simulink model "Encoder_Zynq_V25"  (R2021a)
settings: Solver=FixedStepDiscrete  StartTime=0.0  StopTime=SimulationsDauer  RelTol=1e-3
values from neighbouring files (symbols this model uses):
  f_ISR = 40e3    (= 40000)    [Script_Encoder_Zynq.m]
  IncPerTurn = 1024    [Script_Encoder_Zynq.m]
  inital_zero_speed_timeout = speed_timeout_in_s*f_fpga    (= 10000)    [Script_Encoder_Zynq.m]
  n_max = 6000    [Script_Encoder_Zynq.m]
  OmegaPerOverSampl = 500*((2*pi)/60)    (= 52.3598775598)    [Script_Encoder_Zynq.m]
  Periode = abs(1/Striche_pro_Sekunde)    [Script_Encoder_Zynq.m]
  Phase_Delay_A = Periode/8    [Script_Encoder_Zynq.m]
  Phase_Delay_B = -Periode/8    [Script_Encoder_Zynq.m]
  PolePair = 1    [Script_Encoder_Zynq.m]
  QuadratureFactor = 4    [Script_Encoder_Zynq.m]
  reciprocal_iterations = 3    [Script_Encoder_Zynq.m]
  T_50MHz = 1/f_50MHz    (= 1e-08)    [Script_Encoder_Zynq.m]
  T_mech = 1e-08    [Script_Encoder_Zynq.m]
undefined symbols (not defined in the file or in its folder): DiscIntNeverNeededParam, Newton, Raphson
libraries: hdlsllib x17, dspsrcs4 x3, simulink x2, dspswit3 x2, spsEdgeDetectorLib x2, simulink_extras x1, spspowerguiLib x1
(part 1 of 3)
settings Model: DataTypeOverride=Off  Creator=Wendel_ELSYS  LastModifiedBy=ga92wum
settings SolverCC: ConcurrentTasks=on  AlgebraicLoopSolver=TrustRegion  MinimalZcImpactIntegration=on
settings DataIOCC: LimitDataPoints=on  SaveFormat=Array
settings OptimizationCC: BlockReduction=off  ConditionallyExecuteInputs=off  DefaultParameterBehavior=Inlined  LifeSpan=inf
settings DebuggingCC: ReadBeforeWriteMsg=DisableAll  WriteAfterWriteMsg=DisableAll  WriteAfterReadMsg=DisableAll  AlgebraicLoopMsg=error  SingleTaskRateTransMsg=error  ParameterOverflowMsg=none  SFUnexpectedBacktrackingDiag=warning  SFNoUnconditionalDefaultTransitionDiag=warning  SFExecutionAtInitializationDiag=none  SFMachineParentedDataDiag=warning  ArithmeticOperatorsInVariantConditions=warning
settings HardwareCC: ProdBitPerPointer=32  ProdBitPerSizeT=32  ProdBitPerPtrDiffT=32  ProdLargestAtomicFloat=None  ProdIntDivRoundTo=Undefined  ProdEndianess=Unspecified  ProdWordSize=32  ProdHWDeviceType=ASIC/FPGA->ASIC/FPGA  ProdEqTarget=off
settings ModelReferenceCC: UpdateModelReferenceTargets=IfOutOfDate  PropagateSignalLabelsOutOfModel=off
settings SFSimCC: SFSimEcho=off  SimUseLocalCustomCode=off  CustomCodeUndefinedFunction=UseInterfaceOnly
settings RTWCC: RTWUseLocalCustomCode=off
settings CodeAppCC: StateflowObjectComments=on
settings GRTTargetCC: TargetLangStandard=C89/C90 (ANSI)
settings ConfigComp: CovMetricSettings=dw  CovSaveCumulativeToWorkspaceVar=on  CovSaveSingleToWorkspaceVar=on  CovExternalEMLEnable=off
settings SimscapeCC: SimscapeNormalizeSystem=off

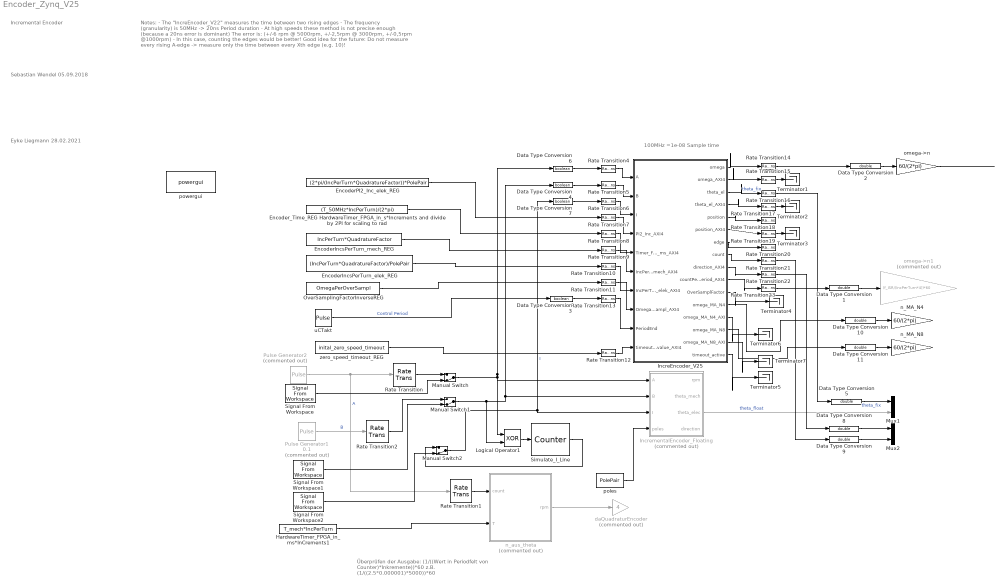
== system Encoder_Zynq_V25 ==
  note: 100MHz =1e-08 Sample time
  note: Überprüfen der Ausgabe:
      | (1/((Wert in Periodfelt von Counter)*Inkremente))*60
      | z.B. (1/((2.5*0.000001)*5000))*60
  note: Sebastian Wendel
      | 05.09.2018
  note: Notes:
      | - The "IncreEncoder_V22" measures the time between two rising edges
      | - The frequency (granularity) is 50MHz -> 20ns Period duration
      | - At high speeds these method is not precise enough (because a 20ns error is dominant)
      | The error is: (+/-6 rpm @ 5000rpm, +/-2,5rpm @ 3000rpm, +/-0,5rpm @1000rpm)
      | - In this case, counting the edges would be better!
      |
      | Good idea for the future: Do not measure every rising A-edge
      | -> measure only the time between every Xth edge (e.g. 10)!
  note: Incremental Encoder
  note: Eyke Liegmann
      | 28.02.2021
  Data Type Conversion{1..2,5,8..11} (7 alike) : DataTypeConversion  OutDataTypeStr=double
  Data Type Conversion{3..4,6..7} (4 alike) : DataTypeConversion  OutDataTypeStr=boolean
  "EncoderIncsPerTurn_elek_REG " : Constant  Value=(IncPerTurn*QuadratureFactor)/PolePair  OutDataTypeStr=fixdt(0,16,0)  SampleTime=T_mech
  EncoderIncsPerTurn_mech_REG : Constant  Value=IncPerTurn*QuadratureFactor  OutDataTypeStr=fixdt(0,16,0)  SampleTime=T_mech
  EncoderPI2_Inc_elek_REG : Constant  Value=(2*pi/(IncPerTurn*QuadratureFactor))*PolePair  OutDataTypeStr=fixdt(0,24,24)  SampleTime=T_mech
  Encoder_Time_REG HardwareTimer_FPGA_in_s*Increments and divide by 2PI for scaling to rad : Constant  Value=(T_50MHz*IncPerTurn)/(2*pi)  OutDataTypeStr=fixdt(0,32,32)  SampleTime=T_mech
  HardwareTimer_FPGA_in_ms*InCrements1 : Constant  Value=T_mech*IncPerTurn  OutDataTypeStr=double  SampleTime=T_mech
  IncreEncoder_V25 : Subsystem  TreatAsAtomicUnit=on
  IncrementalEncoder_Floating : Subsystem  Commented=on
  Logical Operator1 : Logic  Operator=XOR  AllPortsSameDT=off  OutDataTypeStr=boolean
  Manual Switch : ManualSwitch  CurrentSetting=0
  Manual Switch1 : ManualSwitch  CurrentSetting=0
  Manual Switch2 : ManualSwitch  CurrentSetting=0
  Mux1 : Mux  Inputs=2
  Mux2 : Mux  Inputs=2
  OverSamplingFactorInverseREG : Constant  Value=OmegaPerOverSampl  OutDataTypeStr=fixdt(1,24,11)  SampleTime=T_mech
  Pulse Generator1 0.1 : DiscretePulseGenerator  Commented=on  PulseType=Time based  Period=Periode  PulseWidth=50  PhaseDelay=Phase_Delay_B  SampleTime=T_mech  VectorParams1D=off
  Pulse Generator2 : DiscretePulseGenerator  Commented=on  PulseType=Time based  Period=Periode  PulseWidth=50  PhaseDelay=Phase_Delay_A  SampleTime=T_mech  VectorParams1D=off
  Rate Transition{,1..2,14..23} (13 alike) : RateTransition  Deterministic=off  OutPortSampleTime=T_mech
  Rate Transition{4..13} (10 alike) : RateTransition  Deterministic=off  OutPortSampleTime=T_50MHz
  Signal From Workspace : dspsrcs4/Signal From Workspace  X=A_ila  Ts=T_mech  nsamps=1  OutputAfterFinalValue=Setting to zero  ignoreOrWarnInputAndFrameLengths=off  OutputFrames=off
  Signal From Workspace1 : dspsrcs4/Signal From Workspace  X=B_ila  Ts=T_mech  nsamps=1  OutputAfterFinalValue=Setting to zero  ignoreOrWarnInputAndFrameLengths=off  OutputFrames=off
  Signal From Workspace2 : dspsrcs4/Signal From Workspace  X=I_ila  Ts=T_mech  nsamps=1  OutputAfterFinalValue=Setting to zero  ignoreOrWarnInputAndFrameLengths=off  OutputFrames=off
  Simulate_I_Line : dspswit3/Counter  Direction=Up  CountEvent=Either edge  CounterSize=User defined  MaxCount=IncPerTurn*4  InitialCount=0  Output=Hit  HitValue=IncPerTurn*4  ResetInput=off  SamplesPerFrame=1  Ts=1  CntDtype=double  HitDtype=Boolean
  Terminator{1..7} (7 alike) : Terminator
  "daQuadraturEncoder " : Gain  Commented=on  Gain=4
  n_MA_N4 : Gain  Gain=60/(2*pi)  OutDataTypeStr=double
  n_MA_N8 : Gain  Gain=60/(2*pi)  OutDataTypeStr=double
  n_aus_theta : Subsystem  Commented=on  TreatAsAtomicUnit=on
  omega->n : Gain  Gain=60/(2*pi)  OutDataTypeStr=double
  omega->n1 : Gain  Commented=on  Gain=(f_ISR/(IncPerTurn*4))*60  OutDataTypeStr=double
  poles : Constant  Value=PolePair  OutDataTypeStr=uint8  SampleTime=T_mech
  powergui : spspowerguiLib/powergui  Priority=1  SimulationMode=Discrete  SampleTime=T_mech  frequency=60  Iterations=50  frequencyindice=0  Pbase=100e6  ErrMax=1e-4  UnitsV=kV  UnitsW=MW  buscounter=0  FunctionMessages=off  echomessages=off  EnableUseOfTLC=off  CurrentSourceSwitches=off  DisableSnubberDevices=off  DisableRonSwitches=off  DisableVfSwitches=off  DisplayEquations=off  AutomaticDiscreteSolvers=off  SolverType=Tustin  Interpol=off  ExternalGateDelay=off  methode=off  Ts=0  x0status=blocks  SPID=off  SwTol=0  HookPort=off  NonlinearTolerance=1e-4  nMaxIteration=100  ContinueOnMaxIteration=off  RestoreLinks=warning  ResistiveCurrentMeasurement=off  Frange=[0:2:500]  Ylog=off  Xlog=on  ShowGrid=off  save=off  variable=ZData  structure=0  ZoomFFT=on  StartTime=0.0  cycles=1  DisplayStyle=1  fundamental=60  FreqAxis=off  MaxFrequency=1000  frequencyindicesteady=1  RmsSteady=1  display=off
  uCTakt : DiscretePulseGenerator  PulseType=Time based  Period=1/f_ISR  PulseWidth=f_ISR*T_50MHz *100  SampleTime=T_mech  VectorParams1D=off
  zero_speed_timeout_REG : Constant  Value=inital_zero_speed_timeout  OutDataTypeStr=uint32  SampleTime=T_mech
  wires:
  Pulse Generator1 0.1/1 -> Rate Transition2/1  "B"
  Manual Switch1/1 -> Logical Operator1/2, Data Type Conversion4/1, IncrementalEncoder_Floating/2(B)
  Manual Switch2/1 -> Data Type Conversion7/1, IncrementalEncoder_Floating/3(I)  "I"
  Logical Operator1/1 -> Simulate_I_Line/1
  Manual Switch/1 -> Data Type Conversion6/1, IncrementalEncoder_Floating/1(A), Logical Operator1/1
  Data Type Conversion6/1 -> Rate Transition4/1
  Data Type Conversion4/1 -> Rate Transition5/1
  Data Type Conversion7/1 -> Rate Transition6/1
  IncreEncoder_V25/1(omega) -> Rate Transition14/1
  IncreEncoder_V25/9(direction_AXI4) -> Rate Transition22/1
  IncreEncoder_V25/7(edge) -> Rate Transition20/1
  IncreEncoder_V25/8(count) -> Rate Transition21/1
  IncrementalEncoder_Floating/3(theta_elec) -> Mux1/2  "theta_float"
  poles/1 -> IncrementalEncoder_Floating/4(poles)
  EncoderPI2_Inc_elek_REG/1 -> Rate Transition7/1
  IncreEncoder_V25/3(theta_el) -> Rate Transition16/1  "theta_fix"
  IncreEncoder_V25/5(position) -> Rate Transition18/1
  IncreEncoder_V25/4(theta_el_AXI4) -> Rate Transition17/1
  IncreEncoder_V25/2(omega_AXI4) -> Rate Transition15/1
  Encoder_Time_REG HardwareTimer_FPGA_in_s*Increments and divide by 2PI for scaling to rad/1 -> Rate Transition8/1
  EncoderIncsPerTurn_mech_REG/1 -> Rate Transition9/1
  "EncoderIncsPerTurn_elek_REG "/1 -> Rate Transition10/1
  omega->n/1 -> ?
  Data Type Conversion2/1 -> omega->n/1
  HardwareTimer_FPGA_in_ms*InCrements1/1 -> n_aus_theta/2(T)
  Rate Transition1/1 -> n_aus_theta/1(count)
  n_aus_theta/1(rpm) -> "daQuadraturEncoder "/1
  Pulse Generator2/1 -> Rate Transition/1, Rate Transition1/1  "A"
  OverSamplingFactorInverseREG/1 -> Rate Transition11/1
  Rate Transition2/1 -> Manual Switch1/1
  Rate Transition/1 -> Manual Switch/1
  uCTakt/1 -> Data Type Conversion3/1  "Control Period"
  Data Type Conversion1/1 -> omega->n1/1
  IncreEncoder_V25/10(countPerPeriod_AXI4) -> Rate Transition23/1
  Data Type Conversion3/1 -> Rate Transition13/1
  IncreEncoder_V25/6(position_AXI4) -> Rate Transition19/1
  Data Type Conversion5/1 -> Mux1/1  "theta_fix"
  Rate Transition4/1 -> IncreEncoder_V25/1(A)
  Rate Transition5/1 -> IncreEncoder_V25/2(B)
  Rate Transition6/1 -> IncreEncoder_V25/3(I)
  Rate Transition7/1 -> IncreEncoder_V25/4(PI2_Inc_AXI4)
  Rate Transition8/1 -> IncreEncoder_V25/5(Timer_FPGA_ms_AXI4)
  Rate Transition9/1 -> IncreEncoder_V25/6(IncPerTurn_mech_AXI4)
  Rate Transition10/1 -> IncreEncoder_V25/7(IncPerTurn_elek_AXI4)
  Rate Transition11/1 -> IncreEncoder_V25/8(OmegaPerOverSampl_AXI4)
  Rate Transition13/1 -> IncreEncoder_V25/9(PeriodEnd)
  Rate Transition14/1 -> Data Type Conversion2/1
  Rate Transition15/1 -> Terminator1/1
  Rate Transition16/1 -> Data Type Conversion5/1
  Rate Transition17/1 -> Terminator2/1
  Rate Transition19/1 -> Terminator3/1
  Rate Transition21/1 -> Data Type Conversion9/1
  Rate Transition22/1 -> Data Type Conversion8/1
  Rate Transition23/1 -> Data Type Conversion1/1
  Data Type Conversion8/1 -> Mux2/1
  Data Type Conversion9/1 -> Mux2/2
  IncreEncoder_V25/11(OverSamplFactor) -> Terminator4/1
  Signal From Workspace/1 -> Manual Switch/2
  Signal From Workspace1/1 -> Manual Switch1/2
  Signal From Workspace2/1 -> Manual Switch2/2
  Simulate_I_Line/1 -> Manual Switch2/1
  IncreEncoder_V25/12(omega_MA_N4) -> Data Type Conversion10/1
  IncreEncoder_V25/13(omega_MA_N4_AXI) -> Terminator6/1
  IncreEncoder_V25/15(omega_MA_N8_AXI) -> Terminator7/1
  Data Type Conversion10/1 -> n_MA_N4/1
  Data Type Conversion11/1 -> n_MA_N8/1
  IncreEncoder_V25/14(omega_MA_N8) -> Data Type Conversion11/1
  Rate Transition12/1 -> IncreEncoder_V25/10(timeout_value_AXI4)
  zero_speed_timeout_REG/1 -> Rate Transition12/1
  IncreEncoder_V25/16(timeout_active) -> Terminator5/1

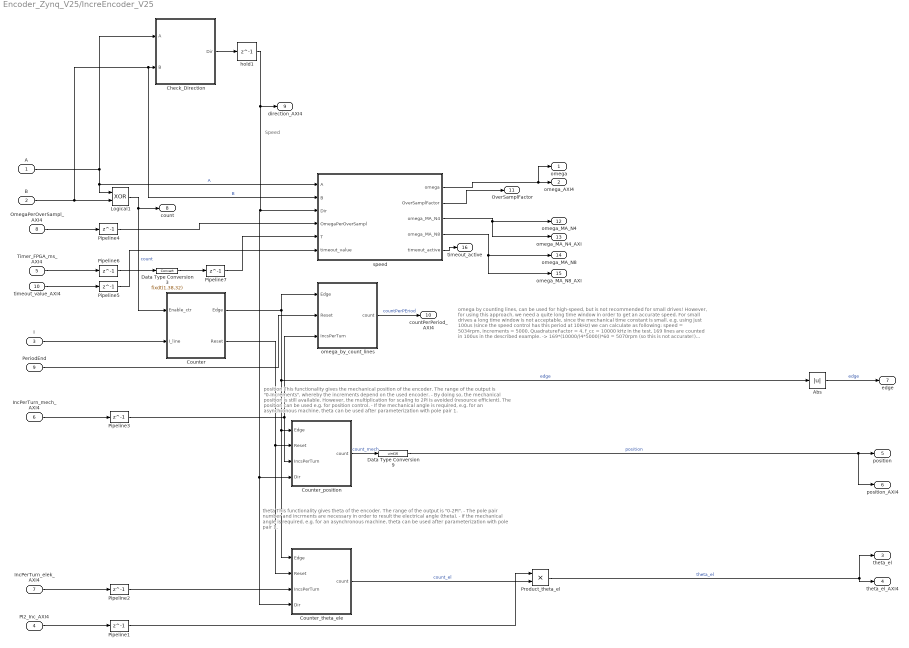
== system Encoder_Zynq_V25/IncreEncoder_V25 ==
  note: omega by counting lines, can be used for high-speed, but is not recommended for small drives!
      | However, for using this approach, we need a quite long time window in order to get an accurate speed.
      | For small drives a long time window is not acceptable, since the mechanical time constant is small.
      | e.g. using just 100us (since the speed control has this period at 10kHz) we can calculate as following:
      | speed = 5034rpm, Increments = 5000, QuadratureFactor = 4, f_cc = 10000 kHz
      | In the test, 169 lines are counted in 100us in the described example.
      | -> 169*(10000/(4*5000))*60 = 5070rpm (so this is not accurate!)
      | However, a longer time window is not acceptabel for speed control with10kHz. More increments is not common, since 5000 are already a lot!
  note: Speed
  note: position
      | This functionality gives the mechanical position of the encoder. The range of the output is "0-Increments", whereby the increments depend on the used encoder.
      | - By doing so, the mechanical position is still available. However, the multiplication for scaling to 2PI is avoided (resource efficient). The position can be used e.g. for position control.
      | - If the mechanical angle is required, e.g. for an asynchronous machine, theta can be used after parameterization with pole pair 1.
  note: theta
      | This functionality gives theta of the encoder. The range of the output is "0-2PI".
      | - The pole pair number and incrments are necessary in order to result the electrical angle (theta).
      | - If the mechanical angle is required, e.g. for an asynchronous machine, theta can be used after parameterization with pole pair 1.
  A : Inport
  B : Inport  Port=2
  I : Inport  Port=3
  PI2_Inc_AXI4 : Inport  Port=4
  Timer_FPGA_ms_AXI4 : Inport  Port=5
  IncPerTurn_mech_AXI4 : Inport  Port=6
  IncPerTurn_elek_AXI4 : Inport  Port=7
  OmegaPerOverSampl_AXI4 : Inport  Port=8
  PeriodEnd : Inport  Port=9
  timeout_value_AXI4 : Inport  Port=10  OutDataTypeStr=uint32
  Abs : Abs  OutDataTypeStr=fixdt(0,1,0)  RndMeth=Simplest
  Check_Direction : Subsystem  TreatAsAtomicUnit=on
  Counter : Subsystem  TreatAsAtomicUnit=on
  Counter_position : Subsystem  TreatAsAtomicUnit=on
  Counter_theta_ele : Subsystem  TreatAsAtomicUnit=on
  Data Type Conversion3 : DataTypeConversion  OutDataTypeStr=fixdt(1,38,32)
  Data Type Conversion9 : DataTypeConversion  OutDataTypeStr=uint16
  Logical1 : Logic  Operator=XOR  AllPortsSameDT=off  OutDataTypeStr=boolean
  Pipeline{1..7} (7 alike) : Delay  DelayLength=1
  Product_theta_el : Product  OutMin=[0]  OutMax=[2*pi]  OutDataTypeStr=fixdt(1,24,20)
  hold1 : Delay  DelayLength=1
  omega_by_count_lines : Subsystem  TreatAsAtomicUnit=on
  speed : Subsystem
  omega : Outport  VectorParamsAs1DForOutWhenUnconnected=off
  omega_AXI4 : Outport  Port=2  VectorParamsAs1DForOutWhenUnconnected=off
  theta_el : Outport  Port=3  VectorParamsAs1DForOutWhenUnconnected=off
  theta_el_AXI4 : Outport  Port=4  VectorParamsAs1DForOutWhenUnconnected=off
  position : Outport  Port=5  VectorParamsAs1DForOutWhenUnconnected=off
  position_AXI4 : Outport  Port=6  VectorParamsAs1DForOutWhenUnconnected=off
  edge : Outport  Port=7  VectorParamsAs1DForOutWhenUnconnected=off
  count : Outport  Port=8  VectorParamsAs1DForOutWhenUnconnected=off
  direction_AXI4 : Outport  Port=9  VectorParamsAs1DForOutWhenUnconnected=off
  countPerPeriod_AXI4 : Outport  Port=10  VectorParamsAs1DForOutWhenUnconnected=off
  OverSamplFactor : Outport  Port=11  VectorParamsAs1DForOutWhenUnconnected=off
  omega_MA_N4 : Outport  Port=12  VectorParamsAs1DForOutWhenUnconnected=off
  omega_MA_N4_AXI : Outport  Port=13  VectorParamsAs1DForOutWhenUnconnected=off
  omega_MA_N8 : Outport  Port=14  VectorParamsAs1DForOutWhenUnconnected=off
  omega_MA_N8_AXI : Outport  Port=15  VectorParamsAs1DForOutWhenUnconnected=off
  timeout_active : Outport  Port=16  OutDataTypeStr=boolean  VectorParamsAs1DForOutWhenUnconnected=off
  wires:
  A/1 -> Check_Direction/1(A), Logical1/1, speed/1(A)  "A"
  B/1 -> speed/2(B), Check_Direction/2(B), Logical1/2  "B"
  I/1 -> Counter/2(I_line)
  hold1/1 -> Counter_theta_ele/4(Dir), Counter_position/4(Dir), speed/3(Dir), direction_AXI4/1
  Counter_position/1(count) -> Data Type Conversion9/1  "count_mech"
  Data Type Conversion9/1 -> position_AXI4/1, position/1  "position"
  Logical1/1 -> Counter/1(Enable_ctr), count/1  "count"
  IncPerTurn_mech_AXI4/1 -> Pipeline3/1
  IncPerTurn_elek_AXI4/1 -> Pipeline2/1
  PI2_Inc_AXI4/1 -> Pipeline1/1
  Counter_theta_ele/1(count) -> Product_theta_el/2  "count_el"
  Product_theta_el/1 -> theta_el/1, theta_el_AXI4/1  "theta_el"
  Timer_FPGA_ms_AXI4/1 -> Pipeline6/1
  Counter/2(Reset) -> Counter_theta_ele/2(Reset), Counter_position/2(Reset)
  Counter/1(Edge) -> Counter_theta_ele/1(Edge), Counter_position/1(Edge), Abs/1, omega_by_count_lines/1(Edge)  "edge"
  Check_Direction/1(Dir) -> hold1/1
  OmegaPerOverSampl_AXI4/1 -> Pipeline4/1
  PeriodEnd/1 -> omega_by_count_lines/2(Reset)
  omega_by_count_lines/1(count) -> countPerPeriod_AXI4/1  "countPerPEriod"
  Abs/1 -> edge/1  "edge"
  Pipeline1/1 -> Product_theta_el/1
  Pipeline2/1 -> Counter_theta_ele/3(IncsPerTurn)
  Pipeline3/1 -> omega_by_count_lines/3(IncsPerTurn), Counter_position/3(IncsPerTurn)
  Pipeline6/1 -> Data Type Conversion3/1
  Data Type Conversion3/1 -> Pipeline7/1
  Pipeline4/1 -> speed/4(OmegaPerOverSampl)
  Pipeline7/1 -> speed/5(T)
  speed/1(omega) -> omega/1, omega_AXI4/1
  speed/2(OverSamplFactor) -> OverSamplFactor/1
  speed/3(omega_MA_N4) -> omega_MA_N4_AXI/1, omega_MA_N4/1
  speed/4(omega_MA_N8) -> omega_MA_N8_AXI/1, omega_MA_N8/1
  timeout_value_AXI4/1 -> Pipeline5/1
  speed/5(timeout_active) -> timeout_active/1
  Pipeline5/1 -> speed/6(timeout_value)

== system Encoder_Zynq_V25/IncrementalEncoder_Floating ==
  A : Inport
  B : Inport  Port=2
  I : Inport  Port=3
  poles : Inport  Port=4
  Add : Sum  Inputs=+-  OutDataTypeStr=fixdt(1,16,0)
  Counter3 : dspswit3/Counter  Direction=Up  CountEvent=Either edge  CounterSize=User defined  MaxCount=IncPerTurn*4  InitialCount=0  Output=Count  HitValue=32  ResetInput=on  SamplesPerFrame=1  Ts=1  CntDtype=double  HitDtype=Logical
  CutTheta_0_2PI : Subsystem
  Edge Detector2 : spsEdgeDetectorLib/Edge Detector  model=Rising  ic=0  Ts=-1
      settings: SourceProductBaseCode=PS
  Edge Detector3 : spsEdgeDetectorLib/Edge Detector  model=Rising  ic=0  Ts=-1
      settings: SourceProductBaseCode=PS
  Logical Operator1 : Logic  Operator=XOR  AllPortsSameDT=off  OutDataTypeStr=boolean
  Logical Operator3 : Logic  AllPortsSameDT=off  OutDataTypeStr=boolean
  Logical Operator4 : Logic  Operator=NOT  AllPortsSameDT=off  OutDataTypeStr=boolean
  Logical Operator5 : Logic  AllPortsSameDT=off  OutDataTypeStr=boolean
  Logical Operator6 : Logic  Operator=NOT  AllPortsSameDT=off  OutDataTypeStr=boolean
  Product : Product
  S-R Flip-Flop1 : simulink_extras/Flip Flops/S-R Flip-Flop  initial_condition=0
  Scope1 : Scope  NumInputPorts=4
  cut_theta_2pi : Gain  Gain=(2*pi)/(IncPerTurn*QuadratureFactor)
  cut_theta_2pi1 : Gain  Gain=(2*pi)/(IncPerTurn*QuadratureFactor)
  n_aus_theta_v4 : Subsystem
  rpm : Outport  VectorParamsAs1DForOutWhenUnconnected=off
  theta_mech : Outport  Port=2  VectorParamsAs1DForOutWhenUnconnected=off
  theta_elec : Outport  Port=3  VectorParamsAs1DForOutWhenUnconnected=off
  direction : Outport  Port=4  VectorParamsAs1DForOutWhenUnconnected=off
  wires:
  I/1 -> Counter3/2
  Counter3/1 -> Product/1, cut_theta_2pi/1, Scope1/1
  n_aus_theta_v4/1(n) -> rpm/1
  Logical Operator1/1 -> Scope1/4, Counter3/1
  cut_theta_2pi/1 -> Scope1/2, n_aus_theta_v4/1(theta), theta_mech/1
  Product/1 -> cut_theta_2pi1/1
  poles/1 -> Product/2
  cut_theta_2pi1/1 -> CutTheta_0_2PI/1(In1)
  CutTheta_0_2PI/1(Out1) -> theta_elec/1
  Edge Detector2/1 -> Logical Operator3/1
  Logical Operator4/1 -> Logical Operator3/2
  Logical Operator3/1 -> S-R Flip-Flop1/1
  Edge Detector3/1 -> Logical Operator5/1
  Logical Operator6/1 -> Logical Operator5/2
  Logical Operator5/1 -> S-R Flip-Flop1/2
  S-R Flip-Flop1/1 -> Add/1
  S-R Flip-Flop1/2 -> Add/2
  A/1 -> Logical Operator6/1, Edge Detector2/1, Logical Operator1/1
  B/1 -> Edge Detector3/1, Logical Operator4/1, Logical Operator1/2
  Add/1 -> direction/1

== system Encoder_Zynq_V25/n_aus_theta ==
  count : Inport
  T : Inport  Port=2
  1/rps->1/omega : Gain  Gain=1/(2*pi)  OutDataTypeStr=double
  Add : Sum  Inputs=+-
  Add1 : Sum
  Constant : Constant  Value=0  OutDataTypeStr=double  SampleTime=-1
  Constant1 : Constant  Value=0  OutDataTypeStr=double  SampleTime=-1
  Constant2 : Constant  Value=0  OutDataTypeStr=double  SampleTime=-1
  Divide1 : Product  Inputs=/
  ProtectOverflow_T_count : Switch  Threshold=50
  ProtectOverflow_rps : Switch  Threshold=50  OutDataTypeStr=double
  Scope1 : Scope  NumInputPorts=4
  Scope2 : Scope  NumInputPorts=4
  T_count : Delay  DelayLength=1
  T_count_switch : Switch  Criteria=u2 ~= 0
  count_old : Delay  DelayLength=1
  count_old_switch : Switch  Criteria=u2 ~= 0
  speed_old : Delay  DelayLength=1
  speed_old_switch : Switch  Criteria=u2 ~= 0
  rpm : Outport  VectorParamsAs1DForOutWhenUnconnected=off
  wires:
  count_old_switch/1 -> count_old/1
  count_old/1 -> count_old_switch/3, Add/2
  Constant/1 -> T_count_switch/1
  Add/1 -> speed_old_switch/2, count_old_switch/2, Scope1/1, T_count_switch/2
  Constant1/1 -> ProtectOverflow_T_count/1
  ProtectOverflow_rps/1 -> 1/rps->1/omega/1, Scope2/1
  Constant2/1 -> ProtectOverflow_rps/1
  speed_old_switch/1 -> ProtectOverflow_rps/3, Scope2/3, speed_old/1
  speed_old/1 -> speed_old_switch/3
  T/1 -> Scope2/4, Add1/1
  ProtectOverflow_T_count/1 -> T_count/1
  T_count/1 -> Scope1/4, Add1/2
  Add1/1 -> Scope2/2, speed_old_switch/1, T_count_switch/3
  count/1 -> Add/1, count_old_switch/1
  T_count_switch/1 -> ProtectOverflow_rps/2, Scope1/2, ProtectOverflow_T_count/2, ProtectOverflow_T_count/3
  1/rps->1/omega/1 -> Divide1/1
  Divide1/1 -> rpm/1

== system Encoder_Zynq_V25/IncreEncoder_V25/Check_Direction ==
  A : Inport
  B : Inport  Port=2
  Add : Sum  Inputs=+-  AccumDataTypeStr=fixdt(1,4,0)  OutDataTypeStr=fixdt(1,4,0)
  Add1 : Sum  Inputs=+-  AccumDataTypeStr=fixdt(1,4,0)  OutDataTypeStr=fixdt(1,4,0)
  Add2 : Sum  AccumDataTypeStr=fixdt(1,4,0)  OutDataTypeStr=fixdt(1,4,0)
  Change : Sum  AccumDataTypeStr=fixdt(1,4,0)  OutDataTypeStr=fixdt(1,4,0)
  Change1 : Delay  DelayLength=1
  Save_Direction : Switch  Criteria=u2 ~= 0  Threshold=0.1  OutDataTypeStr=fixdt(1,4,0)
  T_count_switch : Switch  Threshold=1  OutDataTypeStr=Inherit: Inherit via back propagation
  TrnLeft : Sum  Inputs=+-  AccumDataTypeStr=fixdt(1,4,0)  OutDataTypeStr=fixdt(1,4,0)
  TrnRight : Sum  Inputs=+-  AccumDataTypeStr=fixdt(1,4,0)  OutDataTypeStr=fixdt(1,4,0)
  TurnLeft : Constant  Value=-1  OutDataTypeStr=fixdt(1,4,0)  SampleTime=-1
  TurnRight : Constant  OutDataTypeStr=fixdt(1,4,0)  SampleTime=-1
  count_old : Delay  DelayLength=1
  count_old1 : Delay  DelayLength=1
  count_old2 : Delay  DelayLength=1
  count_old_switch : Switch  Criteria=u2 ~= 0  OutDataTypeStr=Inherit: Inherit via back propagation
  count_old_switch1 : Switch  Criteria=u2 ~= 0  OutDataTypeStr=Inherit: Inherit via back propagation
  new_value : Delay  DelayLength=1
  nothing : Constant  Value=0  OutDataTypeStr=fixdt(1,4,0)  SampleTime=-1
  nothing1 : Constant  Value=0  OutDataTypeStr=fixdt(1,4,0)  SampleTime=-1
  speed_old_switch : Switch  Threshold=1  OutDataTypeStr=Inherit: Inherit via back propagation
  Dir : Outport  VectorParamsAs1DForOutWhenUnconnected=off
  wires:
  A/1 -> TrnLeft/2, Add/1, count_old_switch/1
  count_old_switch/1 -> count_old/1
  count_old/1 -> count_old_switch/3, Add/2
  TurnRight/1 -> T_count_switch/1
  Add/1 -> TrnRight/1, count_old_switch/2  "Edge_A"
  T_count_switch/1 -> Change/1, Add2/1
  Save_Direction/1 -> count_old2/1
  B/1 -> TrnRight/2, Add1/1, count_old_switch1/1
  count_old_switch1/1 -> count_old1/1
  count_old1/1 -> count_old_switch1/3, Add1/2
  Add1/1 -> TrnLeft/1, count_old_switch1/2  "Edge_B"
  TrnRight/1 -> T_count_switch/2  "Trn_Right"
  new_value/1 -> Save_Direction/1
  TrnLeft/1 -> speed_old_switch/2  "TrnLeft"
  TurnLeft/1 -> speed_old_switch/1
  nothing/1 -> speed_old_switch/3
  nothing1/1 -> T_count_switch/3
  speed_old_switch/1 -> Change/2, Add2/2
  Add2/1 -> new_value/1
  Change/1 -> Change1/1
  Change1/1 -> Save_Direction/2  "Change"
  count_old2/1 -> Save_Direction/3, Dir/1  "Dir"

== system Encoder_Zynq_V25/IncreEncoder_V25/Counter ==
  note: 1 for one cycle if edge recognized
  note: Reset
  Enable_ctr : Inport
  I_line : Inport  Port=2
  Detec_edge : Sum  Inputs=+-  AccumDataTypeStr=int8  OutDataTypeStr=int8
  Reset_flag : Sum  Inputs=+-  AccumDataTypeStr=uint8  OutDataTypeStr=uint8
  reset_old : Delay  DelayLength=1
  reset_old1 : Delay  DelayLength=1
  reset_old_switch : Switch  Criteria=u2 ~= 0
  reset_old_switch1 : Switch  Criteria=u2 ~= 0
  Edge : Outport  VectorParamsAs1DForOutWhenUnconnected=off
  Reset : Outport  Port=2  VectorParamsAs1DForOutWhenUnconnected=off
  wires:
  I_line/1 -> Reset_flag/1, reset_old_switch/1
  reset_old_switch/1 -> reset_old/1
  reset_old/1 -> reset_old_switch/3, Reset_flag/2
  Reset_flag/1 -> Reset/1, reset_old_switch/2
  Enable_ctr/1 -> Detec_edge/1, reset_old_switch1/1
  reset_old_switch1/1 -> reset_old1/1
  reset_old1/1 -> reset_old_switch1/3, Detec_edge/2
  Detec_edge/1 -> reset_old_switch1/2, Edge/1  "1 for one cycle if edge recognized"

== system Encoder_Zynq_V25/IncreEncoder_V25/Counter_position ==
  note: Count
  note: Check if count is to big 0-Increments
  note: Check if count is to small
  Edge : Inport
  Reset : Inport  Port=2
  IncsPerTurn : Inport  Port=3
  Dir : Inport  Port=4
  Add1 : Sum  AccumDataTypeStr=int16  OutDataTypeStr=int16
  Constant1 : Constant  Value=0  OutDataTypeStr=int16  SampleTime=-1
  Constant2 : Constant  OutDataTypeStr=int16  SampleTime=-1
  Constant3 : Constant  Value=0  OutDataTypeStr=int16  SampleTime=-1
  Constant5 : Constant  Value=-1  OutDataTypeStr=int16  SampleTime=-1
  Relational Operator : RelationalOperator  Operator=>  OutDataTypeStr=boolean  RndMeth=Nearest
  Relational Operator1 : RelationalOperator  Operator=<=  OutDataTypeStr=boolean  RndMeth=Nearest
  Resett_switch1 : Switch  Criteria=u2 ~= 0  OutDataTypeStr=uint16
  Resett_switch2 : Switch  Criteria=u2 ~= 0  OutDataTypeStr=int16
  Resett_switch3 : Switch  Criteria=u2 ~= 0  OutDataTypeStr=int16
  only_use_for_neg_speed : Switch  Threshold=1
  reset_old{1..6} (6 alike) : Delay  DelayLength=1
  speed_old_switch1 : Switch  Criteria=u2 ~= 0
  speed_old_switch2 : Switch  Threshold=1
  count : Outport  VectorParamsAs1DForOutWhenUnconnected=off
  wires:
  Reset/1 -> Resett_switch2/2
  Edge/1 -> speed_old_switch1/2  "1 for one cycle if edge recognized"
  Add1/1 -> Resett_switch2/3
  speed_old_switch1/1 -> Add1/1
  Constant3/1 -> speed_old_switch1/3
  Constant2/1 -> speed_old_switch2/1
  Dir/1 -> reset_old6/1
  Constant5/1 -> speed_old_switch2/3
  speed_old_switch2/1 -> reset_old4/1
  Relational Operator/1 -> reset_old3/1
  Constant1/1 -> Resett_switch1/1, only_use_for_neg_speed/1, Relational Operator1/2, Resett_switch2/1
  Resett_switch2/1 -> Resett_switch3/3
  Resett_switch3/1 -> Relational Operator1/1, Resett_switch1/3
  Relational Operator1/1 -> reset_old2/1
  only_use_for_neg_speed/1 -> Resett_switch3/2
  reset_old4/1 -> speed_old_switch1/1
  IncsPerTurn/1 -> reset_old5/1
  reset_old6/1 -> only_use_for_neg_speed/2, speed_old_switch2/2
  Resett_switch1/1 -> Relational Operator/1, reset_old1/1, count/1
  reset_old3/1 -> Resett_switch1/2
  reset_old2/1 -> only_use_for_neg_speed/3
  reset_old5/1 -> Relational Operator/2, Resett_switch3/1
  reset_old1/1 -> Add1/2

== system Encoder_Zynq_V25/IncreEncoder_V25/Counter_theta_ele ==
  note: This Reset (I-Line) synchronize only
      | theta with position.
      | Since I-Line comes only once per
      | mechanical turn. Normaly the "IncsPerTurn"
      | do the Reset.
  note: Count
  note: Check if count is to big
      | -Count from 0-Increments
      | - e.g. for 5000 increments, 4 pole pairs and A/B-Line (quadrature),
      | we count from 0-(5000*4/4) = 0-5000
      | - In that case, we must reset to 0, as soon as we have a value,
      | which is 1 bigger than increments (e.g. 5001 = 0).
  note: Check if count is to small
  Edge : Inport
  Reset : Inport  Port=2
  IncsPerTurn : Inport  Port=3
  Dir : Inport  Port=4
  Add1 : Sum  AccumDataTypeStr=int16  OutDataTypeStr=int16
  Constant1 : Constant  Value=0  OutDataTypeStr=int16  SampleTime=-1
  Constant2 : Constant  OutDataTypeStr=int16  SampleTime=-1
  Constant3 : Constant  Value=0  OutDataTypeStr=int16  SampleTime=-1
  Constant5 : Constant  Value=-1  OutDataTypeStr=int16  SampleTime=-1
  Relational Operator : RelationalOperator  Operator=>  OutDataTypeStr=boolean  RndMeth=Nearest
  Relational Operator1 : RelationalOperator  Operator=<=  OutDataTypeStr=boolean  RndMeth=Nearest
  Reset_switch3 : Switch  Criteria=u2 ~= 0  OutDataTypeStr=int16
  Resett_switch1 : Switch  Criteria=u2 ~= 0  OutDataTypeStr=int16
  Resett_switch2 : Switch  Criteria=u2 ~= 0  OutDataTypeStr=int16
  only_use_for_neg_speed : Switch  Threshold=1
  reset_old{1..6} (6 alike) : Delay  DelayLength=1
  speed_old_switch1 : Switch  Criteria=u2 ~= 0
  speed_old_switch2 : Switch  Threshold=1
  count : Outport  VectorParamsAs1DForOutWhenUnconnected=off
  wires:
  Reset/1 -> Resett_switch2/2
  Edge/1 -> speed_old_switch1/2  "1 for one cycle if edge recognized"
  Add1/1 -> Resett_switch2/3
  speed_old_switch1/1 -> Add1/1
  Constant3/1 -> speed_old_switch1/3
  Constant2/1 -> speed_old_switch2/1
  IncsPerTurn/1 -> reset_old1/1
  Dir/1 -> reset_old5/1
  Constant5/1 -> speed_old_switch2/3
  speed_old_switch2/1 -> reset_old4/1
  Resett_switch1/1 -> reset_old6/1, count/1, Relational Operator/1
  Relational Operator/1 -> reset_old3/1
  Constant1/1 -> Resett_switch2/1, only_use_for_neg_speed/1, Relational Operator1/2, Resett_switch1/1
  Resett_switch2/1 -> Reset_switch3/3
  Reset_switch3/1 -> Relational Operator1/1, Resett_switch1/3
  Relational Operator1/1 -> reset_old2/1
  only_use_for_neg_speed/1 -> Reset_switch3/2
  reset_old4/1 -> speed_old_switch1/1
  reset_old5/1 -> speed_old_switch2/2, only_use_for_neg_speed/2
  reset_old3/1 -> Resett_switch1/2
  reset_old2/1 -> only_use_for_neg_speed/3
  reset_old1/1 -> Relational Operator/2, Reset_switch3/1
  reset_old6/1 -> Add1/2

== system Encoder_Zynq_V25/IncreEncoder_V25/omega_by_count_lines ==
  note: Set new counter value
  note: Check if count is to big in order to safe for value overflow
  note: Count
  Edge : Inport
  Reset : Inport  Port=2
  IncsPerTurn : Inport  Port=3
  Add1 : Sum  AccumDataTypeStr=int16  OutDataTypeStr=int16
  Constant1 : Constant  Value=0  OutDataTypeStr=int16  SampleTime=-1
  Constant2 : Constant  OutDataTypeStr=int16  SampleTime=-1
  Constant3 : Constant  Value=0  OutDataTypeStr=int16  SampleTime=-1
  Constant4 : Constant  Value=10  OutDataTypeStr=int16  SampleTime=-1
  Relational Operator : RelationalOperator  Operator=>  OutDataTypeStr=boolean  RndMeth=Nearest
  Reset_when_overflow : Sum  OutDataTypeStr=int16
  Resett_switch1 : Switch  Criteria=u2 ~= 0  OutDataTypeStr=int16
  Resett_switch2 : Switch  Criteria=u2 ~= 0  OutDataTypeStr=int16
  reset_old{1,3..5} (4 alike) : Delay  DelayLength=1
  reset_old_switch1 : Switch  Criteria=u2 ~= 0
  speed_old_switch1 : Switch  Criteria=u2 ~= 0
  count : Outport  VectorParamsAs1DForOutWhenUnconnected=off
  wires:
  Reset_when_overflow/1 -> reset_old5/1
  Relational Operator/1 -> Resett_switch1/2
  speed_old_switch1/1 -> Add1/1
  reset_old5/1 -> Relational Operator/2
  Resett_switch2/1 -> Resett_switch1/3
  reset_old4/1 -> speed_old_switch1/1
  Edge/1 -> speed_old_switch1/2  "1 for one cycle if edge recognized"
  Constant1/1 -> Resett_switch2/1, Resett_switch1/1
  Constant3/1 -> speed_old_switch1/3
  IncsPerTurn/1 -> Reset_when_overflow/2
  Add1/1 -> Resett_switch2/3
  Constant2/1 -> reset_old4/1
  Constant4/1 -> Reset_when_overflow/1
  Resett_switch1/1 -> reset_old3/1
  reset_old3/1 -> reset_old_switch1/1, Add1/2, Relational Operator/1
  reset_old1/1 -> reset_old_switch1/3
  Reset/1 -> reset_old_switch1/2, Resett_switch2/2  "Use new value"
  reset_old_switch1/1 -> reset_old1/1, count/1

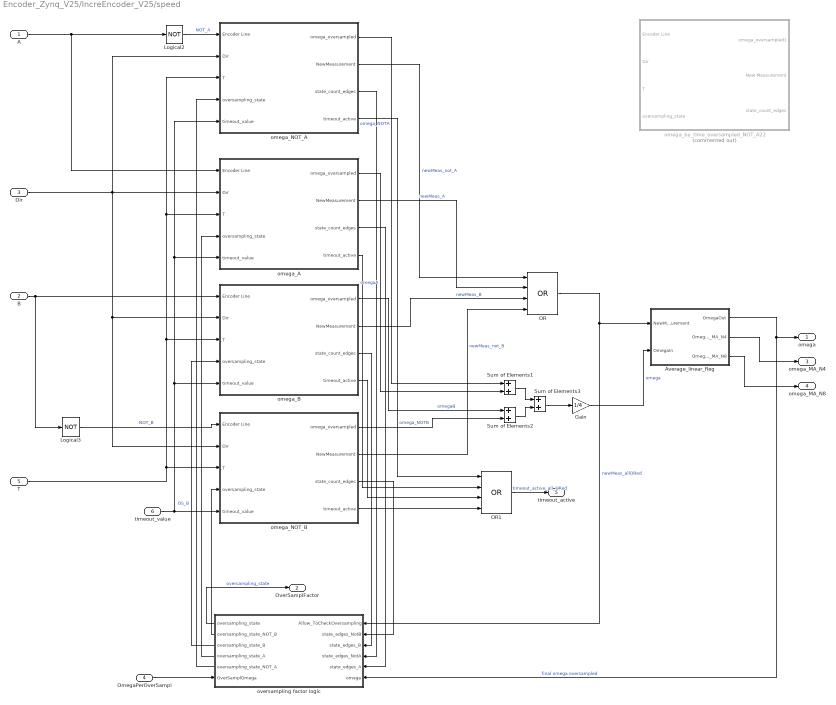
== system Encoder_Zynq_V25/IncreEncoder_V25/speed ==
  A : Inport
  B : Inport  Port=2
  Dir : Inport  Port=3
  OmegaPerOverSampl : Inport  Port=4
  T : Inport  Port=5
  timeout_value : Inport  Port=6  OutDataTypeStr=uint32
  Average_linear_Reg : Subsystem
  Gain : Gain  Gain=1/4  OutDataTypeStr=Inherit: Same as input
  Logical2 : Logic  Operator=NOT  AllPortsSameDT=off  OutDataTypeStr=boolean
  Logical3 : Logic  Operator=NOT  AllPortsSameDT=off  OutDataTypeStr=boolean
  OR : Logic  Operator=OR  Inputs=4  IconShape=distinctive  AllPortsSameDT=off  OutDataTypeStr=boolean
  OR1 : Logic  Operator=OR  Inputs=4  IconShape=distinctive  AllPortsSameDT=off  OutDataTypeStr=boolean
  Sum of Elements1 : Sum  Inputs=2
  Sum of Elements2 : Sum  Inputs=2
  Sum of Elements3 : Sum  Inputs=2
  omega_A : Subsystem  TreatAsAtomicUnit=on
  omega_B : Subsystem  TreatAsAtomicUnit=on
  omega_NOT_A : Subsystem  TreatAsAtomicUnit=on
  omega_NOT_B : Subsystem  TreatAsAtomicUnit=on
  omega_by_time_oversampled_NOT_A22 : Subsystem  Commented=on
  oversampling factor logic : Subsystem
      settings: PortSchema="{\"entries\":[{\"content\":{\"sides\":[{\"content\":{\"connectorIds\":[\"In1\",\"In2\",\"In3\",\"In4\",\"In5\",\"In6\"]},\"type\":\"ConnectorPlacement.EquallySpacedRectSide\",\"uuid\":\"00190a63-1990-4dc8-8561-af6346041cd2\"},{\"content\":{\"connectorIds\":[\"Out1\",\"Out2\",\"Out3\",\"Out4\",\"Out5\",\"In7\"],\"side\":\"RIGHT\"},\"type\":\"ConnectorPlacement.EquallySpacedRectSide\",\"uuid\":\"ed8fa1bb-ba76-4f60-9676-d72d7f094a86\"},{\"content\":{\"connectorIds\":[],\"side\":\"TOP\"},\"type\":\"ConnectorPlacement.EquallySpacedRectSide\",\"uuid\":\"16aa4cab-6298-4523-a92b-d078d21511a0\"}]},\"type\":\"ConnectorPlacement.EquallySpacedConnector\",\"uuid\":\"bb0c721d-662f-49b4-b1e3-cc7ff0334cdb\"}],\"packageUris\":[\"http://schema.mathworks.com/mf0/Connector/R2020b\"],\"version\":\"1.0\"}"
  omega : Outport  VectorParamsAs1DForOutWhenUnconnected=off
  OverSamplFactor : Outport  Port=2
  omega_MA_N4 : Outport  Port=3  VectorParamsAs1DForOutWhenUnconnected=off
  omega_MA_N8 : Outport  Port=4  VectorParamsAs1DForOutWhenUnconnected=off
  timeout_active : Outport  Port=5  OutDataTypeStr=boolean  VectorParamsAs1DForOutWhenUnconnected=off
  wires:
  Logical3/1 -> omega_NOT_B/1(Encoder Line)  "NOT_B"
  T/1 -> omega_NOT_B/3(T), omega_B/3(T), omega_NOT_A/3(T), omega_A/3(T)
  Dir/1 -> omega_NOT_B/2(Dir), omega_B/2(Dir), omega_A/2(Dir), omega_NOT_A/2(Dir)
  Logical2/1 -> omega_NOT_A/1(Encoder Line)  "NOT_A"
  B/1 -> Logical3/1, omega_B/1(Encoder Line)
  A/1 -> omega_A/1(Encoder Line), Logical2/1
  Sum of Elements3/1 -> Gain/1
  omega_A/1(omega_oversampled) -> Sum of Elements1/2  "omegaA"
  Gain/1 -> Average_linear_Reg/2("OmegaIn ")  "omega"
  omega_NOT_B/1(omega_oversampled) -> Sum of Elements2/2  "omega_NOTB"
  omega_B/1(omega_oversampled) -> Sum of Elements2/1  "omegaB"
  omega_NOT_A/1(omega_oversampled) -> Sum of Elements1/1  "omega_NOTA"
  omega_NOT_B/2(NewMeasurement) -> OR/4  "newMeas_not_B"
  omega_B/2(NewMeasurement) -> OR/3  "newMeas_B"
  omega_A/2(NewMeasurement) -> OR/2  "newMeas_A"
  omega_NOT_A/2(NewMeasurement) -> OR/1  "newMeas_not_A"
  Average_linear_Reg/1(OmegaOut) -> oversampling factor logic/6(omega), omega/1  "final omega oversampled"
  OmegaPerOverSampl/1 -> oversampling factor logic/7(OverSamplOmega)
  OR/1 -> oversampling factor logic/1(Allow_ToCheckOversampling), Average_linear_Reg/1(NewMeasurement)  "newMeas_allORed"
  oversampling factor logic/1(oversampling_state) -> OverSamplFactor/1  "oversampling_state"
  omega_B/3(state_count_edges) -> oversampling factor logic/3(state_edges_B)
  omega_A/3(state_count_edges) -> oversampling factor logic/5(state_edges_A)
  omega_NOT_A/3(state_count_edges) -> oversampling factor logic/4(state_edges_NotA)
  oversampling factor logic/4(oversampling_state_A) -> omega_A/4(oversampling_state)
  oversampling factor logic/2(oversampling_state_NOT_B) -> omega_NOT_B/4(oversampling_state)
  oversampling factor logic/3(oversampling_state_B) -> omega_B/4(oversampling_state)  "OS_B"
  oversampling factor logic/5(oversampling_state_NOT_A) -> omega_NOT_A/4(oversampling_state)
  omega_NOT_B/3(state_count_edges) -> oversampling factor logic/2(state_edges_NotB)
  Average_linear_Reg/2(OmegaOut_MA_N4) -> omega_MA_N4/1
  Average_linear_Reg/3(OmegaOut_MA_N8) -> omega_MA_N8/1
  omega_NOT_B/4(timeout_active) -> OR1/4
  timeout_value/1 -> omega_A/5(timeout_value), omega_NOT_A/5(timeout_value), omega_B/5(timeout_value), omega_NOT_B/5(timeout_value)
  OR1/1 -> timeout_active/1  "timeout_active_all_ORed"
  omega_B/4(timeout_active) -> OR1/3
  omega_A/4(timeout_active) -> OR1/2
  omega_NOT_A/4(timeout_active) -> OR1/1
  Sum of Elements2/1 -> Sum of Elements3/2
  Sum of Elements1/1 -> Sum of Elements3/1

== system Encoder_Zynq_V25/IncrementalEncoder_Floating/CutTheta_0_2PI ==
  In1 : Inport
  Add7 : Sum  Inputs=+-  OutDataTypeStr=double
  Gain : Gain  Gain=1/(2*pi)
  Gain11 : Gain  Gain=2*pi
  Rounding Function : Rounding
  Out1 : Outport  VectorParamsAs1DForOutWhenUnconnected=off
  wires:
  Gain/1 -> Rounding Function/1
  Rounding Function/1 -> Gain11/1
  Gain11/1 -> Add7/2
  In1/1 -> Gain/1, Add7/1
  Add7/1 -> Out1/1

== system Encoder_Zynq_V25/IncrementalEncoder_Floating/n_aus_theta_v4 ==
  theta : Inport
  Abs : Abs
  Add : Sum  Inputs=-+
  Add1 : Sum  Inputs=+-
  Gain : Gain  Gain=2*pi
  Gain1 : Gain  Gain=1/T_mech
  Gain2 : Gain  Gain=60/(2*pi)
  Geschwindigkeitsfilter1 : Subsystem
  Rate Limiter2 1/T : RateLimiter  RisingSlewLimit=1/T_mech*10  FallingSlewLimit=-1/T_mech*10  SampleTimeMode=inherited
  Saturation : Saturate  UpperLimit=n_max  LowerLimit=-n_max
  Scope1 : Scope  NumInputPorts=5
  Scope2 : Scope  NumInputPorts=5
  Sign : Signum
  Switch : Switch  Threshold=3
  Unit Delay : UnitDelay  SampleTime=-1  HasFrameUpgradeWarning=on
  n : Outport  VectorParamsAs1DForOutWhenUnconnected=off
  wires:
  Switch/1 -> Scope1/3, Gain1/1
  Add/1 -> Scope2/1, Switch/1
  Gain/1 -> Add/1
  Sign/1 -> Gain/1
  Add1/1 -> Scope2/3, Add/2, Abs/1, Scope2/2, Switch/3, Sign/1
  Abs/1 -> Scope1/4, Switch/2
  Gain1/1 -> Scope1/2, Gain2/1
  theta/1 -> Scope2/5, Add1/1, Unit Delay/1
  Unit Delay/1 -> Scope2/4, Add1/2
  Gain2/1 -> Saturation/1
  Geschwindigkeitsfilter1/1(Out1) -> Scope1/5, Rate Limiter2 1/T/1
  Rate Limiter2 1/T/1 -> n/1
  Saturation/1 -> Scope1/1, Geschwindigkeitsfilter1/1(In1)

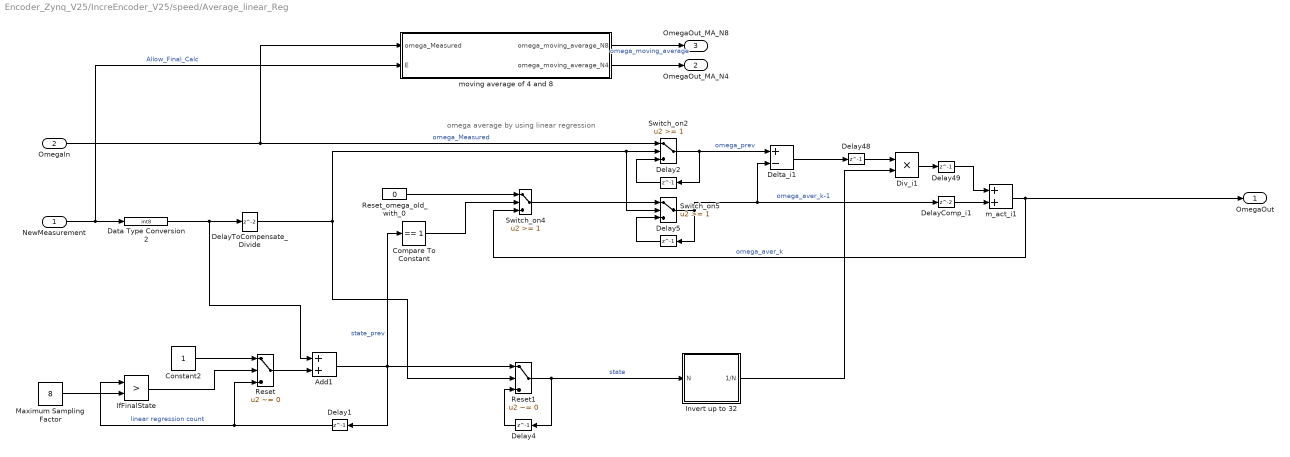
== system Encoder_Zynq_V25/IncreEncoder_V25/speed/Average_linear_Reg ==
  note: omega average by using linear regression
  NewMeasurement : Inport
  "OmegaIn " : Inport  Port=2
  Add1 : Sum  OutDataTypeStr=Inherit: Same as accumulator
  Compare To Constant : simulink/Logic and Bit Operations/Compare To Constant  relop===  const=1  OutDataTypeStr=boolean
  Constant2 : Constant  OutDataTypeStr=int8  SampleTime=T_50MHz
  Data Type Conversion2 : DataTypeConversion  OutDataTypeStr=int8
  Delay{1..2,4..5,48..49} (6 alike) : Delay  DelayLength=1  InitialCondition=0
  DelayComp_i1 : Delay  InitialCondition=0
  DelayToCompensate_Divide : Delay
  Delta_i1 : Sum  Inputs=+-  AccumDataTypeStr=fixdt(1,32,18)  OutDataTypeStr=fixdt(1,24,11)
  Div_i1 : Product  Inputs=**  RndMeth=Simplest  SaturateOnIntegerOverflow=on  OutDataTypeStr=Inherit: Same as first input
  IfFinalState : RelationalOperator  Operator=>  OutDataTypeStr=boolean  RndMeth=Nearest
  Invert up to 32 : Subsystem
  Maximum Sampling Factor : Constant  Value=8  OutDataTypeStr=int8  SampleTime=T_50MHz
  Reset : Switch  Criteria=u2 ~= 0  Threshold=0.5  OutDataTypeStr=fixdt(1,24,11)
  Reset1 : Switch  Criteria=u2 ~= 0  Threshold=0.5  OutDataTypeStr=fixdt(1,24,11)
  Reset_omega_old_with_0 : Constant  Value=0  OutDataTypeStr=fixdt(1,24,11)  SampleTime=-1
  Switch_on2 : Switch  Threshold=1  OutDataTypeStr=fixdt(1,24,11)  RndMeth=Simplest
  Switch_on4 : Switch  Threshold=1  OutDataTypeStr=Inherit: Inherit via back propagation  RndMeth=Simplest
  Switch_on5 : Switch  Threshold=1  OutDataTypeStr=Inherit: Inherit via back propagation  RndMeth=Simplest
  m_act_i1 : Sum  OutDataTypeStr=Inherit: Same as accumulator  RndMeth=Simplest
  moving average of 4 and 8 : Subsystem
  OmegaOut : Outport  VectorParamsAs1DForOutWhenUnconnected=off
  OmegaOut_MA_N4 : Outport  Port=2  VectorParamsAs1DForOutWhenUnconnected=off
  OmegaOut_MA_N8 : Outport  Port=3  VectorParamsAs1DForOutWhenUnconnected=off
  wires:
  Maximum Sampling Factor/1 -> IfFinalState/2
  Compare To Constant/1 -> Switch_on4/2
  DelayToCompensate_Divide/1 -> Reset1/2, Switch_on5/2, Switch_on2/2
  Delay4/1 -> Reset1/3
  Reset1/1 -> Delay4/1, Invert up to 32/1(N)  "state"
  Switch_on4/1 -> Switch_on5/1
  Reset_omega_old_with_0/1 -> Switch_on4/1
  Delay1/1 -> Reset/3, IfFinalState/1  "linear regression count"
  Data Type Conversion2/1 -> DelayToCompensate_Divide/1, Add1/1
  Constant2/1 -> Reset/1
  Reset/1 -> Add1/2
  IfFinalState/1 -> Reset/2
  Add1/1 -> Compare To Constant/1, Delay1/1, Reset1/1  "state_prev"
  Delay2/1 -> Switch_on2/3
  Switch_on2/1 -> Delta_i1/1, Delay2/1  "omega_prev"
  Div_i1/1 -> Delay49/1
  Delay48/1 -> Div_i1/1
  Delta_i1/1 -> Delay48/1
  Delay49/1 -> m_act_i1/1
  Switch_on5/1 -> Delay5/1, Delta_i1/2, DelayComp_i1/1  "omega_aver_k-1"
  m_act_i1/1 -> OmegaOut/1, Switch_on4/3  "omega_aver_k"
  "OmegaIn "/1 -> moving average of 4 and 8/1(omega_Measured), Switch_on2/1  "omega_Measured"
  DelayComp_i1/1 -> m_act_i1/2
  NewMeasurement/1 -> moving average of 4 and 8/2(E), Data Type Conversion2/1  "Allow_Final_Calc"
  Delay5/1 -> Switch_on5/3
  Invert up to 32/1(1/N) -> Div_i1/2
  moving average of 4 and 8/2(omega_moving_average_N4) -> OmegaOut_MA_N4/1
  moving average of 4 and 8/1(omega_moving_average_N8) -> OmegaOut_MA_N8/1  "omega_moving_average"

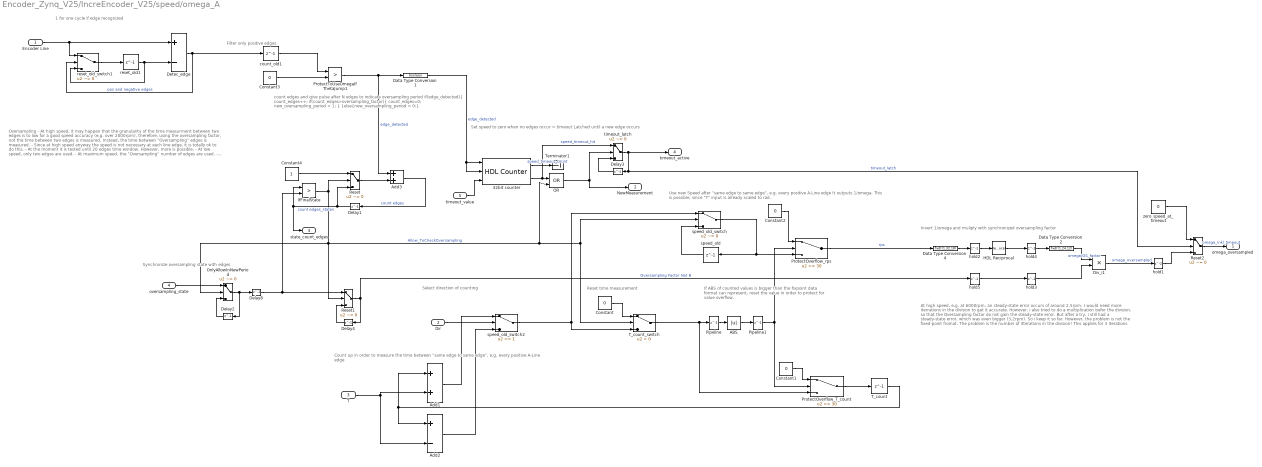
== system Encoder_Zynq_V25/IncreEncoder_V25/speed/omega_A ==
  note: Oversampling
      | - At high speed, it may happen that the granularity of the time measurment between
      | two edges is to low for a good speed accuracy (e.g. over 2000rpm), therefore, using
      | the oversampling factor, not the time between two edges is measured. Instead, the
      | time between "Oversampling" edges is measured.
      | - Since at high speed anyway the speed is not necessary at each line edge,
      |  it is totally ok to do this.
      | - At the moment it is tested until 20 edges time window. However, more is possible.
      | - At low speed, only two edges are used.
      | - At maximum speed, the "Oversampling" number of edges are used.
      | - Between them, a linear factor is used.
      | - Using the OverSampling number also at low speed is not possible,
      |  since the fixpoint range must be quite high! (fixdt(1,36,30) is used at the moment)
  note: Count up in order to measure the time between "same edge to same edge", e.g. every positive A-Line edge
  note: Reset time measurement
  note: 1 for one cycle if edge recognized
  note: Use new Speed after "same edge to same edge", e.g. every positive A-Line edge
      | It outputs 1/omega. This is possible, since "T" input is already scaled to rad.
  note: Select direction of counting
  note: If ABS of counted values is bigger than the
      | fixpoint data format can represent, reset the
      | value in order to protect for value overflow.
  note: Filter only positive edges
  note: count edges and give pulse after N edges to indicate oversampling period
      | if(edge_detected){
      | 	count_edges++;
      | 	if(count_edges>oversampling_factor){
      | 		count_edges=0;
      | 		new_oversampling_period = 1;
      | 	}
      | }else{new_oversampling_period = 0;}
  note: Synchronize oversampling state with edges
  note: At high speed, e.g. at 6000rpm, an steady-state error occurs of around 2.5rpm. I would need more iterrations in the division to get it accurate.
      | However, i also tried to do a multiplication befor the division, so that the Oversampling factor do not gain the steady-state error.
      | But after a try, i still had a steady-state error, which was even bigger (3,2rpm). So i keep it so far.
      | However, the problem is not the fixed-point fromat. The problem is the number of itterations in the division!
      | This applies for 3 iterations
  note: Invert 1/omega and muliply with synchronized oversampling factor
  note: Set speed to zero when no edges occur = timeout
      | Latched until a new edge occurs
  Encoder Line : Inport
  Dir : Inport  Port=2
  T : Inport  Port=3
  oversampling_state : Inport  Port=4
  timeout_value : Inport  Port=5  OutDataTypeStr=uint32
  32bit counter : hdlsllib/Sources/HDL Counter  CountType=Count limited  CountInit=0  CountStep=1  CountMax=inital_zero_speed_timeout  CountFromType=Initial value  CountFrom=0  CountResetPort=on  CountLoadPort=on  CountEnbPort=off  CountDirPort=off  CountHitOutputPort=on  CountDataType=Unsigned  CountWordLen=32  CountFracLen=0  CountSampTime=1
  ABS : Abs
  Add1 : Sum  OutDataTypeStr=Inherit: Same as first input
  Add2 : Sum  Inputs=+-  OutDataTypeStr=Inherit: Same as first input
  Add3 : Sum  OutDataTypeStr=Inherit: Same as accumulator
  Constant : Constant  Value=0  OutDataTypeStr=fixdt(1,38,32)  SampleTime=-1
  Constant1 : Constant  Value=0  OutDataTypeStr=fixdt(1,38,32)  SampleTime=-1
  Constant2 : Constant  Value=0  OutDataTypeStr=fixdt(1,38,32)  SampleTime=-1
  Constant3 : Constant  Value=0  OutDataTypeStr=int8  SampleTime=-1
  Constant4 : Constant  OutDataTypeStr=int8  SampleTime=T_50MHz
  Data Type Conversion1 : DataTypeConversion  OutDataTypeStr=boolean
  Data Type Conversion2 : DataTypeConversion  OutDataTypeStr=fixdt(1,24,12)
  Data Type Conversion4 : DataTypeConversion  OutDataTypeStr=fixdt(1,32,18)
  Delay{1..4,8} (5 alike) : Delay  DelayLength=1  InitialCondition=0
  Detec_edge : Sum  Inputs=+-  AccumDataTypeStr=int8  OutDataTypeStr=int8
  Div_i1 : Product  Inputs=**  OutDataTypeStr=fixdt(1,24,11)  RndMeth=Simplest  SaturateOnIntegerOverflow=on
  HDL Reciprocal : Reciprocal  NumberOfIterations=reciprocal_iterations
  IfFinalState : RelationalOperator  Operator=>  OutDataTypeStr=boolean  RndMeth=Nearest
  OR : Logic  Operator=OR  IconShape=distinctive  AllPortsSameDT=off  OutDataTypeStr=boolean
  OnlyAllowInNewPeriod : Switch  Criteria=u2 ~= 0  Threshold=0.5  OutDataTypeStr=fixdt(0,16,0)
  Pipeline : Delay  DelayLength=1
  Pipeline1 : Delay  DelayLength=1
  ProtectOverflow_T_count : Switch  Threshold=30
  ProtectOverflow_rps : Switch  Threshold=30  OutDataTypeStr=fixdt(1,38,32)
  ProtectToUseOmegaIfThetaJump1 : RelationalOperator  Operator=>  OutDataTypeStr=fixdt(1,16)  RndMeth=Nearest
  Reset : Switch  Criteria=u2 ~= 0  Threshold=0.5  OutDataTypeStr=fixdt(1,24,11)
  Reset1 : Switch  Criteria=u2 ~= 0  Threshold=0.5  OutDataTypeStr=Inherit: Inherit via back propagation
  Reset2 : Switch  Criteria=u2 ~= 0  Threshold=0.5  OutDataTypeStr=Inherit: Inherit via back propagation
  T_count : Delay  DelayLength=1
  T_count_switch : Switch  Criteria=u2 > Threshold
  Terminator1 : Terminator
  count_old1 : Delay  DelayLength=1
  hold1 : Delay
  hold{2..5} (4 alike) : Delay  DelayLength=1
  reset_old1 : Delay  DelayLength=1
  reset_old_switch1 : Switch  Criteria=u2 ~= 0
  speed_old : Delay  DelayLength=1
  speed_old_switch : Switch  Criteria=u2 ~= 0  OutDataTypeStr=fixdt(1,38,32)
  speed_old_switch2 : Switch  Threshold=1
  timeout_latch : Switch  Criteria=u2 ~= 0  Threshold=0.5  OutDataTypeStr=Inherit: Inherit via back propagation
  zero_speed_at_timeout : Constant  Value=0  OutDataTypeStr=fixdt(1,24,12)  SampleTime=-1
  omega_oversampled : Outport  VectorParamsAs1DForOutWhenUnconnected=off
  NewMeasurement : Outport  Port=2  VectorParamsAs1DForOutWhenUnconnected=off
  state_count_edges : Outport  Port=3  VectorParamsAs1DForOutWhenUnconnected=off
  timeout_active : Outport  Port=4  OutDataTypeStr=boolean  VectorParamsAs1DForOutWhenUnconnected=off
  wires:
  Constant/1 -> T_count_switch/1
  Constant1/1 -> ProtectOverflow_T_count/1
  Constant2/1 -> ProtectOverflow_rps/1
  speed_old_switch/1 -> ProtectOverflow_rps/3, speed_old/1
  speed_old/1 -> speed_old_switch/3
  T/1 -> Add1/2, Add2/2
  ProtectOverflow_T_count/1 -> T_count/1
  T_count/1 -> Add2/1, Add1/1
  speed_old_switch2/1 -> speed_old_switch/1, T_count_switch/3
  count_old1/1 -> ProtectToUseOmegaIfThetaJump1/1
  Constant3/1 -> ProtectToUseOmegaIfThetaJump1/2
  Encoder Line/1 -> reset_old_switch1/1, Detec_edge/1
  reset_old_switch1/1 -> reset_old1/1
  reset_old1/1 -> reset_old_switch1/3, Detec_edge/2
  Detec_edge/1 -> reset_old_switch1/2, count_old1/1  "pos and negative edges"
  Dir/1 -> speed_old_switch2/2
  Add1/1 -> speed_old_switch2/1
  Add2/1 -> speed_old_switch2/3
  T_count_switch/1 -> Pipeline/1, ProtectOverflow_T_count/3
  ABS/1 -> Pipeline1/1
  Pipeline/1 -> ABS/1
  Pipeline1/1 -> ProtectOverflow_T_count/2, ProtectOverflow_rps/2
  IfFinalState/1 -> OR/2, speed_old_switch/2, T_count_switch/2, Reset1/2, OnlyAllowInNewPeriod/2, Reset/2  "Allow_ToCheckOversampling"
  OnlyAllowInNewPeriod/1 -> Delay2/1, Delay8/1
  Delay1/1 -> Reset/3, state_count_edges/1, IfFinalState/1  "count edges_states"
  Add3/1 -> Delay1/1  "count edges"
  Reset/1 -> Add3/2
  Constant4/1 -> Reset/1
  Reset1/1 -> Delay4/1, hold5/1  "Oversampling Factor Not B"
  Delay2/1 -> OnlyAllowInNewPeriod/3
  oversampling_state/1 -> OnlyAllowInNewPeriod/1
  Delay4/1 -> Reset1/3
  Delay8/1 -> Reset1/1, IfFinalState/2
  ProtectToUseOmegaIfThetaJump1/1 -> Add3/1, Data Type Conversion1/1  "edge_detected"
  32bit counter/2 -> OR/1, timeout_latch/1  "speed_timeout_hit"
  OR/1 -> NewMeasurement/1, timeout_latch/2
  Div_i1/1 -> hold1/1  "omega_oversampled"
  hold2/1 -> HDL Reciprocal/1
  hold4/1 -> Data Type Conversion2/1
  HDL Reciprocal/1 -> hold4/1
  hold5/1 -> hold3/1
  hold3/1 -> Div_i1/2
  Data Type Conversion2/1 -> Div_i1/1  "omega/OS_factor"
  ProtectOverflow_rps/1 -> Data Type Conversion4/1  "rps"
  Data Type Conversion4/1 -> hold2/1
  zero_speed_at_timeout/1 -> Reset2/1
  Reset2/1 -> omega_oversampled/1  "omega_inkl_timeout"
  timeout_latch/1 -> timeout_active/1, Reset2/2, Delay3/1  "timeout_latch"
  Delay3/1 -> timeout_latch/3
  Data Type Conversion1/1 -> 32bit counter/2, 32bit counter/1  "edge_detected"
  timeout_value/1 -> 32bit counter/3
  32bit counter/1 -> Terminator1/1  "speed_timeout_count"
  hold1/1 -> Reset2/3
